simulink model "EMPlanner_cs"  (R2020a)
settings: Solver=ode5  StartTime=0.0  StopTime=55  FixedStep=1/1000  RelTol=1e-3
PreLoadFcn:
  | mbxruntime.callbacks.PreLoadFcn(bdroot);
PostLoadFcn:
  | mbxruntime.callbacks.PostLoadFcn(bdroot);
InitFcn:
  | mbxruntime.callbacks.InitFcn(bdroot);
StartFcn:
  | mbxruntime.callbacks.StartFcn(bdroot);
StopFcn:
  | mbxruntime.callbacks.StopFcn(bdroot);
model workspace: external: MAT-File .\EMPlanner_cs_hws.mat (data not in the file)
values from neighbouring files (symbols this model uses):
  c_factor = 43.75    [emplanner_init.m]
  cf = -175016    [emplanner_init.m]
  control_predict_time = 0.01    [emplanner_init.m]
  cr = -130634    [emplanner_init.m]
  dp_col = 4    [emplanner_init.m]
  dp_row = 9    [emplanner_init.m]
  dp_sample_l = 1    [emplanner_init.m]
  dp_sample_s = 15    [emplanner_init.m]
  dp_w_obs = 1e8    (= 100000000)    [emplanner_init.m]
  dp_w_ref = 20    [emplanner_init.m]
  dp_w_smooth_dddl = 10000    [emplanner_init.m]
  dp_w_smooth_ddl = 2000    [emplanner_init.m]
  dp_w_smooth_dl = 300    [emplanner_init.m]
  KD_PID_distance = 0.0    (= 0)    [emplanner_init.m]
  KD_PID_speed = 0    [emplanner_init.m]
  KI_PID_distance = 0.0    (= 0)    [emplanner_init.m]
  KI_PID_speed = 0    [emplanner_init.m]
  KP_PID_distance = 0.5    [emplanner_init.m]
  KP_PID_speed = 1.8    [emplanner_init.m]
  la = 1.265    [emplanner_init.m]
  lb = 2.947-1.265    (= 1.682)    [emplanner_init.m]
  LQR_K1 = k(:,1)'    [emplanner_init.m]
  LQR_K2 = k(:,2)'    [emplanner_init.m]
  LQR_K3 = k(:,3)'    [emplanner_init.m]
  LQR_K4 = k(:,4)'    [emplanner_init.m]
  m = 2020    [emplanner_init.m]
  path_x = [7.7742 8.77358225507 9.77170536558 10.7685522493 11.7641171228 12.7583983581 13.7513958557 14.7431100776 15.7335416918 16.7226914411 17.7105600952 18.6971484329 ... (551 elements, 551x1)]    [test_path.mat]
  path_y = [-207.8202 -207.82020006 -207.820200616 -207.820202023 -207.82020429 -207.820207237 -207.820210603 -207.820214131 -207.82021762 -207.820220941 -207.820224011 -207.820226778 ... (551 elements, 551x1)]    [test_path.mat]
  qp_referenceline_w_length = 2    [emplanner_init.m]
  qp_referenceline_w_ref = 3    [emplanner_init.m]
  qp_referenceline_w_smooth = 1    [emplanner_init.m]
  qp_referenceline_x_lb = -0.2    [emplanner_init.m]
  qp_referenceline_x_ub = 0.2    [emplanner_init.m]
  qp_referenceline_y_lb = -0.2    [emplanner_init.m]
  qp_referenceline_y_ub = 0.2    [emplanner_init.m]
  rack_displacement = [-39.14 , -37.2 , -35.29 , -33.43 , -31.6 , -29.81 , -28.06 , -26.34 , -24.66 ,      -23.01 , -21.38 , -19.79 , -18.23 , -16.69 , -15.18 , -13.7 , -12.23 , -10.8 , -9.38 , -7.98 ,     -6.61 , -5.25 , -3.91 , -2.59 , -1.29 , 0 , 1.27 , 2.54 , 3.78 , 5.02 , 6.24 , 7.46 , 8.66 ,      9.86 , 11.05 , 12.24 , 13.41 , 14.59 , 15.76 , 16.92 , 18.09 , 19.25 , 20.42 , 21.59 , 22.76 ,      23.93 , 25.11 , 26 ...(+26 chars)    [emplanner_init.m]
  right_wheel_ground = [-70 ,-67.2 , -64.4 , -61.6 , -58.8 , -56 , -53.2 , -50.4 , -47.6 , -44.8 , -42 ,      -39.2 , -36.4 , -33.6 , -30.8 , -28 , -25.2 , -22.4 , -19.6 , -16.8 , -14 , -11.2 , -8.4 , -5.6 ,      -2.8 , 0 , 2.8 , 5.6 , 8.4 , 11.2 , 14 , 16.8 , 19.6 , 22.4 , 25.2 , 28 , 30.8 , 33.6 , 36.4 ,      39.2 , 42 , 44.8 , 47.6 , 50.4 , 53.2 , 56 , 58.8 , 61.6 , 64.4 , 67.2 , 70 ]    [emplanner_init.m]
  vx_break_point = zeros(1,5000)    [emplanner_init.m]
undefined symbols (not defined in the file or in its folder): aubr, DiscIntNeverNeededParam, tablebr, vubr, warningInitialVelocity, x0
libraries: simulink x19, PreScanSimulinkLibrary x12, simulink_extras x5, Solver_SF x1
(part 7 of 9)

== system EMPlanner_cs/Audi_A8_Sedan_2/Dynamics_Simple/ShiftLogic/Detect Increase/Other ==
  In1 : Inport
  Action Port : ActionPort  PropagateVarSize=During execution  ActionPortLabel=else
  Data Type Conversion : DataTypeConversion  OutDataTypeStr=double
  Detect Increase : simulink/Logic and Bit Operations/Detect Increase  vinit=0.0  OutDataTypeStr=uint8
  Out1 : Outport
  wires:
  In1/1 -> Detect Increase/1
  Detect Increase/1 -> Data Type Conversion/1
  Data Type Conversion/1 -> Out1/1

== system EMPlanner_cs/Audi_A8_Sedan_2/Dynamics_Simple/Transmission/Transmission_Ratio/If Action Neutral ==
  In1 : Inport
  Action Port : ActionPort  InitializeStates=reset  PropagateVarSize=During execution  ActionPortLabel=if(u1 == 0)
  Out1 : Outport
  wires:
  In1/1 -> Out1/1

== system EMPlanner_cs/Audi_A8_Sedan_2/Dynamics_Simple/Transmission/Transmission_Ratio/If Action Normal ==
  In1 : Inport
  Action Port : ActionPort  InitializeStates=reset  PropagateVarSize=During execution  ActionPortLabel=else
  Out1 : Outport
  wires:
  In1/1 -> Out1/1

== system EMPlanner_cs/Audi_A8_Sedan_2/Dynamics_Simple/Transmission/Transmission_Ratio/If Action Reverse ==
  In1 : Inport
  Action Port : ActionPort  InitializeStates=reset  PropagateVarSize=During execution  ActionPortLabel=elseif(u1 == -1)
  Reverse : Gain  Gain=-1
  Out1 : Outport
  wires:
  Reverse/1 -> Out1/1
  In1/1 -> Reverse/1

== system EMPlanner_cs/Audi_A8_Sedan_2/PathFollower_Preview_1/LateralController/SteeringWheelAngle/FirstOrderDynamics ==
  In : Inport
  TimeConstant[s] : Inport  Port=2
  Reset : Inport  Port=3
  x0 : Inport  Port=4
  1|TimeConstant : Product  Inputs=*/  InputSameDT=on  SaturateOnIntegerOverflow=on  OutDataTypeStr=Inherit: Same as first input
  Discrete-Time Integrator : DiscreteIntegrator  ExternalReset=rising  InitialConditionSource=external  InitialCondition=x0  SampleTime=CSSampleTime  ICPrevOutput=DiscIntNeverNeededParam  ICPrevScaledInput=DiscIntNeverNeededParam
  IC : InitialCondition  Value=0
  Saturation : Saturate  UpperLimit=1e300  LowerLimit=0.001
  Sum : Sum  Inputs=-+|  InputSameDT=on  SaturateOnIntegerOverflow=on  OutDataTypeStr=Inherit: Same as first input
  Out : Outport
  wires:
  IC/1 -> Discrete-Time Integrator/3
  In/1 -> Sum/2
  x0/1 -> IC/1
  Reset/1 -> Discrete-Time Integrator/2
  1|TimeConstant/1 -> Discrete-Time Integrator/1
  Sum/1 -> 1|TimeConstant/1
  Saturation/1 -> 1|TimeConstant/2
  TimeConstant[s]/1 -> Saturation/1
  Discrete-Time Integrator/1 -> Out/1, Sum/1

== system EMPlanner_cs/Audi_A8_Sedan_2/PathFollower_Preview_1/LateralController/SteeringWheelAngle/Sat_Total ==
  In : Inport
  Sat_Limit : Inport  Port=2
  Gain1 : Gain  Gain=-1  SaturateOnIntegerOverflow=on  OutDataTypeStr=Inherit: Same as input  ParamDataTypeStr=Inherit: Same as input
  RelOp_UL : RelationalOperator  RndMeth=Nearest
  RelOp_UL1 : RelationalOperator  Operator=<=  RndMeth=Nearest
  Sum : Sum  Inputs=++|  SaturateOnIntegerOverflow=on
  Switch : Switch  Threshold=0.5  SaturateOnIntegerOverflow=on
  Switch1 : Switch  Threshold=0.5  SaturateOnIntegerOverflow=on
  Sat_Total : Outport
  Sat_Info : Outport  Port=2
  wires:
  Sat_Limit/1 -> Gain1/1, Switch/1, RelOp_UL/2
  RelOp_UL/1 -> Switch/2, Sum/2
  Switch/1 -> RelOp_UL1/1, Switch1/3
  Gain1/1 -> RelOp_UL1/2, Switch1/1
  RelOp_UL1/1 -> Switch1/2, Sum/1
  In/1 -> Switch/3, RelOp_UL/1
  Switch1/1 -> Sat_Total/1
  Sum/1 -> Sat_Info/1

== system EMPlanner_cs/Audi_A8_Sedan_2/PathFollower_Preview_1/LongitudinalController/If Desired Velocity ~= 0/PID_AWU ==
  e : Inport
  Derivative Gain : Gain  Gain=D  SaturateOnIntegerOverflow=on  OutDataTypeStr=Inherit: Same as input  ParamDataTypeStr=Inherit: Same as input
  Discrete-Time Integrator : DiscreteIntegrator  gainval=1  SampleTime=CSSampleTime  UpperSaturationLimit=100  LowerSaturationLimit=-100  ICPrevOutput=DiscIntNeverNeededParam  ICPrevScaledInput=DiscIntNeverNeededParam
  Filter : DiscreteIntegrator  gainval=1  SampleTime=CSSampleTime  ICPrevOutput=DiscIntNeverNeededParam  ICPrevScaledInput=DiscIntNeverNeededParam
  Integral Gain : Gain  Gain=I  SaturateOnIntegerOverflow=on  OutDataTypeStr=Inherit: Same as input  ParamDataTypeStr=Inherit: Same as input
  Integral Gain1 : Gain  Gain=LongCtrl_AWU  SaturateOnIntegerOverflow=on  OutDataTypeStr=Inherit: Same as input  ParamDataTypeStr=Inherit: Same as input
  Proportional Gain : Gain  Gain=P  SaturateOnIntegerOverflow=on  OutDataTypeStr=Inherit: Same as input  ParamDataTypeStr=Inherit: Same as input
  Saturation : Saturate  UpperLimit=100  LowerLimit=-100
  Sum : Sum  Inputs=+++  InputSameDT=on  SaturateOnIntegerOverflow=on  OutDataTypeStr=Inherit: Same as first input
  Sum1 : Sum  Inputs=|+-  InputSameDT=on  SaturateOnIntegerOverflow=on  OutDataTypeStr=Inherit: Same as first input
  Sum2 : Sum  Inputs=|++  InputSameDT=on  SaturateOnIntegerOverflow=on  OutDataTypeStr=Inherit: Same as first input
  Sum3 : Sum  Inputs=-+|  InputSameDT=on  SaturateOnIntegerOverflow=on  OutDataTypeStr=Inherit: Same as first input
  u : Outport  InitialOutput=0
  wires:
  Integral Gain1/1 -> Sum2/2
  Sum3/1 -> Integral Gain1/1
  Saturation/1 -> Sum3/2, u/1
  Sum2/1 -> Discrete-Time Integrator/1
  Sum1/1 -> Sum/3, Filter/1
  Filter/1 -> Sum1/2
  Derivative Gain/1 -> Sum1/1
  Sum/1 -> Sum3/1, Saturation/1
  e/1 -> Integral Gain/1, Proportional Gain/1, Derivative Gain/1
  Discrete-Time Integrator/1 -> Sum/2
  Proportional Gain/1 -> Sum/1
  Integral Gain/1 -> Sum2/1

== system EMPlanner_cs/Audi_A8_Sedan_2/Dynamics_Simple/Chassis/Bicycle_model_[XYZ]/X_Motion/Air&RoadResistance ==
  vx_[ms-1] : Inport
  Gain : Gain  Gain=1/p.Rw
  Road & Aerodyn Resistances : Fcn  Expr=p.Rroad + p.Rair*u^2
  Saturation1 : Saturate  UpperLimit=5/15  LowerLimit=-5/15
  Sign : Signum
  "[ms-1] 2 [rads-1]" : Gain  Gain=1/p.Rw  SaturateOnIntegerOverflow=on  OutDataTypeStr=Inherit: Same as input  ParamDataTypeStr=Inherit: Same as input
  signed load1 : Product  InputSameDT=on  SaturateOnIntegerOverflow=on  OutDataTypeStr=Inherit: Same as first input
  Resistance_Force : Outport
  wires:
  signed load1/1 -> Resistance_Force/1  "F_[N]"
  vx_[ms-1]/1 -> Road & Aerodyn Resistances/1, "[ms-1] 2 [rads-1]"/1
  Saturation1/1 -> Sign/1
  "[ms-1] 2 [rads-1]"/1 -> Saturation1/1
  Road & Aerodyn Resistances/1 -> Gain/1  "ResistanceTorque_[Nm]"
  Sign/1 -> signed load1/2  "sign"
  Gain/1 -> signed load1/1  "Resistance Force_[N]"

== system EMPlanner_cs/Audi_A8_Sedan_2/Dynamics_Simple/Chassis/Bicycle_model_[XYZ]/X_Motion/BrakeSystem ==
  vx_[ms-1] : Inport
  BrakePressure_[bar] : Inport  Port=2
  Gain : Gain  Gain=1/p.Rw
  Saturation : Saturate  UpperLimit=p.PBrakeMax  LowerLimit=0
  Saturation1 : Saturate  UpperLimit=5/15  LowerLimit=-5/15
  Sign : Signum
  "[ms-1] 2 [rads-1]" : Gain  Gain=1/p.Rw  SaturateOnIntegerOverflow=on  OutDataTypeStr=Inherit: Same as input  ParamDataTypeStr=Inherit: Same as input
  braking Q factor : Gain  Gain=p.Qfac  SaturateOnIntegerOverflow=on  OutDataTypeStr=Inherit: Same as input  ParamDataTypeStr=Inherit: Same as input
  signed load1 : Product  InputSameDT=on  SaturateOnIntegerOverflow=on  OutDataTypeStr=Inherit: Same as first input
  BrakeForce : Outport
  BrakeTorqueAbs : Outport  Port=2
  wires:
  braking Q factor/1 -> BrakeTorqueAbs/1, Gain/1
  BrakePressure_[bar]/1 -> Saturation/1
  Saturation/1 -> braking Q factor/1
  vx_[ms-1]/1 -> "[ms-1] 2 [rads-1]"/1
  Saturation1/1 -> Sign/1
  "[ms-1] 2 [rads-1]"/1 -> Saturation1/1
  Sign/1 -> signed load1/2  "sign"
  signed load1/1 -> BrakeForce/1
  Gain/1 -> signed load1/1

== system EMPlanner_cs/Audi_A8_Sedan_2/Dynamics_Simple/Chassis/Bicycle_model_[XYZ]/X_Motion/Configurable Subsystem ==
  In1 : Inport
  In2 : Inport  Port=2
  In3 : Inport  Port=3
  Integrator : Integrator  ExternalReset=level  InitialConditionSource=external
  Out1 : Outport
  wires:
  In1/1 -> Integrator/1
  In2/1 -> Integrator/2
  In3/1 -> Integrator/3
  Integrator/1 -> Out1/1

== system EMPlanner_cs/Audi_A8_Sedan_2/Dynamics_Simple/Chassis/Bicycle_model_[XYZ]/X_Motion/Configurable Subsystem1 ==
  In1 : Inport
  Torsional damping : TransferFcn  Denominator=[0.1 1]
  Out1 : Outport
  wires:
  In1/1 -> Torsional damping/1
  Torsional damping/1 -> Out1/1

== system EMPlanner_cs/Audi_A8_Sedan_2/Dynamics_Simple/Chassis/Bicycle_model_[XYZ]/X_Motion/Max RPM and zero- velocity detection ==
  note: Set to zero after infinite small time-step
  note: Zero velocity detection
  ax : Inport
  Drive Torque : Inport  Port=2
  Brake Torque : Inport  Port=3
  v0 : Inport  Port=4
  vx : Inport  Port=5
  Abs : Abs
  Abs1 : Abs
  Compare To Zero : simulink/Logic and Bit Operations/Compare To Zero  relop=<=  OutDataTypeStr=boolean  ZeroCross=off
  Compare To Zero1 : simulink/Logic and Bit Operations/Compare To Zero  relop=>=  OutDataTypeStr=boolean  ZeroCross=off
  Compare To Zero2 : simulink/Logic and Bit Operations/Compare To Zero  relop=>=  OutDataTypeStr=boolean  ZeroCross=off
  Compare To Zero3 : simulink/Logic and Bit Operations/Compare To Zero  relop=<=  OutDataTypeStr=boolean  ZeroCross=off
  Configurable Subsystem : Subsystem  BlockChoice=Step  mask{ComputationMode=ComputationMode}
      mask prompts: ComputationMode "Compuation mode:"
      mask init:
      | SetComputationMode(gcb,ComputationMode);
      settings: AttributesFormatString=%<BlockChoice>  OpenFcn=BringToFront(gcb);  MemberBlocks=Discrete Step,Step
      settings: TemplateBlock=|
      | PreScanSimulinkLibrary/Configurable Subsystems/Step Function/Configurable
      | Subsystem
  Constant : Constant
  Constant1 : Constant
  Logical Operator : Logic  AllPortsSameDT=off  OutDataTypeStr=boolean
  Logical Operator1 : Logic  AllPortsSameDT=off  OutDataTypeStr=boolean
  Logical Operator2 : Logic  Operator=NOT  AllPortsSameDT=off  OutDataTypeStr=boolean
  Logical Operator3 : Logic  AllPortsSameDT=off  OutDataTypeStr=boolean
  Logical Operator4 : Logic  Operator=OR  AllPortsSameDT=off  OutDataTypeStr=boolean
  Memory : Memory
  Memory1 : Memory
  Memory2 : Memory
  Product : Product  RndMeth=Zero
  Relational Operator : RelationalOperator  Operator=<  OutDataTypeStr=boolean  RndMeth=Nearest
  SR-Memory : Subsystem
  Sum : Sum  Inputs=|-+
  Switch : Switch  Criteria=u2 ~= 0  Threshold=0.5
  ax is 0 : Constant  Value=0
  ax_out : Outport
  vx_reset : Outport  Port=2
  x0 : Outport  Port=3
  wires:
  Logical Operator4/1 -> Logical Operator1/1
  vx/1 -> Compare To Zero/1, Compare To Zero2/1, Memory2/1, Memory/1  "vx"
  Memory2/1 -> Compare To Zero3/1
  Compare To Zero2/1 -> Logical Operator3/1
  Compare To Zero3/1 -> Logical Operator3/2
  Logical Operator3/1 -> Logical Operator4/2  "zero-crossing backward"
  Memory/1 -> Compare To Zero1/1
  Compare To Zero/1 -> Logical Operator/1
  Compare To Zero1/1 -> Logical Operator/2
  Logical Operator/1 -> Logical Operator4/1  "zero-crossing forward"
  Abs/1 -> Relational Operator/1
  Abs1/1 -> Relational Operator/2
  Drive Torque/1 -> Abs/1
  Brake Torque/1 -> Abs1/1
  Relational Operator/1 -> Logical Operator1/2, Logical Operator2/1
  Logical Operator1/1 -> SR-Memory/2(Set)
  Constant/1 -> SR-Memory/1(Signal)
  Logical Operator2/1 -> SR-Memory/3(Reset)
  SR-Memory/1(Out) -> Sum/1, Memory1/1
  Switch/1 -> ax_out/1
  Sum/1 -> Switch/2
  ax is 0/1 -> Switch/3
  Constant1/1 -> Sum/2
  v0/1 -> Product/1
  Product/1 -> x0/1
  Configurable Subsystem/1(Out1) -> Product/2
  ax/1 -> Switch/1  "ax"
  Memory1/1 -> vx_reset/1  "vx"

== system EMPlanner_cs/Audi_A8_Sedan_2/Dynamics_Simple/Chassis/Bicycle_model_[XYZ]/Y & Yaw_Motion/Configurable Subsystem ==
  In1 : Inport
  In2 : Inport  Port=2
  Integrator : Integrator  ExternalReset=level
  Out1 : Outport
  wires:
  In1/1 -> Integrator/1
  In2/1 -> Integrator/2
  Integrator/1 -> Out1/1

== system EMPlanner_cs/Audi_A8_Sedan_2/Dynamics_Simple/Chassis/Bicycle_model_[XYZ]/Y & Yaw_Motion/Configurable Subsystem1 ==
  In1 : Inport
  Integrator : Integrator
  Out1 : Outport
  wires:
  In1/1 -> Integrator/1
  Integrator/1 -> Out1/1

== system EMPlanner_cs/Audi_A8_Sedan_2/Dynamics_Simple/Chassis/Bicycle_model_[XYZ]/Y & Yaw_Motion/Configurable Subsystem2 ==
  In1 : Inport
  In2 : Inport  Port=2
  Integrator : Integrator  ExternalReset=level
  Out1 : Outport
  wires:
  In1/1 -> Integrator/1
  In2/1 -> Integrator/2
  Integrator/1 -> Out1/1

== system EMPlanner_cs/Audi_A8_Sedan_2/Dynamics_Simple/Chassis/Bicycle_model_[XYZ]/Z, Pitch_Motion & Roll_Motion/Configurable Subsystem ==
  In1 : Inport
  Integrator : Integrator  LimitOutput=on  UpperSaturationLimit=5*pi/180  LowerSaturationLimit=-5*pi/180
  Out1 : Outport
  wires:
  In1/1 -> Integrator/1
  Integrator/1 -> Out1/1

== system EMPlanner_cs/Audi_A8_Sedan_2/Dynamics_Simple/Chassis/Bicycle_model_[XYZ]/Z, Pitch_Motion & Roll_Motion/Configurable Subsystem1 ==
  In1 : Inport
  Integrator : Integrator
  Out1 : Outport
  wires:
  In1/1 -> Integrator/1
  Integrator/1 -> Out1/1

== system EMPlanner_cs/Audi_A8_Sedan_2/Dynamics_Simple/Chassis/Bicycle_model_[XYZ]/Z, Pitch_Motion & Roll_Motion/Configurable Subsystem2 ==
  In1 : Inport
  Integrator : Integrator
  Out1 : Outport
  wires:
  In1/1 -> Integrator/1
  Integrator/1 -> Out1/1

== system EMPlanner_cs/Audi_A8_Sedan_2/Dynamics_Simple/Chassis/Bicycle_model_[XYZ]/Z, Pitch_Motion & Roll_Motion/Configurable Subsystem3 ==
  In1 : Inport
  Integrator : Integrator
  Out1 : Outport
  wires:
  In1/1 -> Integrator/1
  Integrator/1 -> Out1/1

== system EMPlanner_cs/Audi_A8_Sedan_2/Dynamics_Simple/Chassis/Bicycle_model_[XYZ]/Z, Pitch_Motion & Roll_Motion/Configurable Subsystem4 ==
  In1 : Inport
  Integrator : Integrator
  Out1 : Outport
  wires:
  In1/1 -> Integrator/1
  Integrator/1 -> Out1/1

== system EMPlanner_cs/Audi_A8_Sedan_2/Dynamics_Simple/Chassis/Bicycle_model_[XYZ]/Z, Pitch_Motion & Roll_Motion/Configurable Subsystem5 ==
  In1 : Inport
  Integrator : Integrator
  Out1 : Outport
  wires:
  In1/1 -> Integrator/1
  Integrator/1 -> Out1/1

== system EMPlanner_cs/Audi_A8_Sedan_2/Dynamics_Simple/Chassis/Bicycle_model_[XYZ]/Z, Pitch_Motion & Roll_Motion/Configurable Subsystem9 ==
  In1 : Inport
  Derivative : Derivative
  Out1 : Outport
  wires:
  In1/1 -> Derivative/1
  Derivative/1 -> Out1/1

== system EMPlanner_cs/Audi_A8_Sedan_2/Dynamics_Simple/Chassis/FrontTyre/AlphaFront/Enabled Subsystem ==
  In : Inport
  Enable : EnablePort  PropagateVarSize=During execution
  AlphaFront : Fcn  Expr=-atan( (u(2)+u(3)*p.a)/u(1) )
  Alpha : Outport  OutputWhenDisabled=reset  InitialOutput=[0]
  wires:
  AlphaFront/1 -> Alpha/1
  In/1 -> AlphaFront/1

== system EMPlanner_cs/Audi_A8_Sedan_2/Dynamics_Simple/Chassis/RearTyre/AlphaRear/Enabled Subsystem ==
  In : Inport
  Enable : EnablePort  PropagateVarSize=During execution
  AlphaRear : Fcn  Expr=-atan( (u(2)-u(3)*p.b)/u(1) )
  Alpha : Outport  OutputWhenDisabled=reset  InitialOutput=[0]
  wires:
  AlphaRear/1 -> Alpha/1
  In/1 -> AlphaRear/1

== system EMPlanner_cs/Audi_A8_Sedan_2/Dynamics_Simple/Chassis/Bicycle_model_[XYZ]/X_Motion/Max RPM and zero- velocity detection/Configurable Subsystem ==
  Step : Step  Time=0.0001  Before=1  After=0  SampleTime=0
  Out1 : Outport
  wires:
  Step/1 -> Out1/1

== system EMPlanner_cs/Audi_A8_Sedan_2/Dynamics_Simple/Chassis/Bicycle_model_[XYZ]/X_Motion/Max RPM and zero- velocity detection/SR-Memory ==
  Signal : Inport
  Set : Inport  Port=2
  Reset : Inport  Port=3
  Constant : Constant  Value=0
  Detect Rise Positive : simulink/Logic and Bit Operations/Detect Rise Positive  vinit=0  OutDataTypeStr=uint8
  Detect Rise Positive1 : simulink/Logic and Bit Operations/Detect Rise Positive  vinit=0  OutDataTypeStr=uint8
  Manual Switch : ManualSwitch
  Manual Switch1 : ManualSwitch
  Switch : Switch  Criteria=u2 ~= 0
  Switch1 : Switch  Criteria=u2 ~= 0
  Unit Delay : UnitDelay  SampleTime=-1  HasFrameUpgradeWarning=on
  Out : Outport
  wires:
  Constant/1 -> Switch1/1
  Switch/1 -> Switch1/3
  Switch1/1 -> Unit Delay/1, Out/1
  Manual Switch1/1 -> Switch1/2
  Reset/1 -> Manual Switch1/2, Detect Rise Positive1/1
  Detect Rise Positive1/1 -> Manual Switch1/1
  Signal/1 -> Switch/1
  Unit Delay/1 -> Switch/3
  Set/1 -> Detect Rise Positive/1, Manual Switch/2
  Detect Rise Positive/1 -> Manual Switch/1
  Manual Switch/1 -> Switch/2

== matlab function EMPlanner_cs/Audi_A8_Sedan_1/decision&planning module/EM Planner/calc plan start info and stitch trajectory ==
  data: pre_planPath_x_set_gcs input; plan_startPoint_x_gcs output; pre_planPath_y_set_gcs input; pre_planPath_heading_set_gcs input; pre_planPath_kappa_set_gcs input; pre_planPath_velocity_set_gcs input; pre_planPath_acceleration_set_gcs input; pre_planPath_time_set input; current_time input; host_x_gcs input; host_y_gcs input; host_heading_gcs input; host_vx_vcs input; host_vy_vcs input; host_ax_vcs input; host_ay_vcs input; plan_startPoint_y_gcs output; plan_startPoint_heading_gcs output; plan_startPoint_kappa_gcs output; plan_startPoint_vx_gcs output; plan_startPoint_vy_gcs output; plan_startPoint_ax_gcs output; plan_startPoint_ay_gcs output; plan_startPoint_time output; stitchPath_x_set_gcs output; stitchPath_y_set_gcs output; stitchPath_heading_set_gcs output; stitchPath_kappa_set_gcs output; stitchPath_velocity_set_gcs output; stitchPath_acceleration_set_gcs output; stitchPath_time_set output; host_dheading_gcs input
function [plan_startPoint_x_gcs,plan_startPoint_y_gcs,plan_startPoint_heading_gcs,plan_startPoint_kappa_gcs, ...
    plan_startPoint_vx_gcs,plan_startPoint_vy_gcs,plan_startPoint_ax_gcs,plan_startPoint_ay_gcs,plan_startPoint_time,...
    stitchPath_x_set_gcs,stitchPath_y_set_gcs,stitchPath_heading_set_gcs,stitchPath_kappa_set_gcs,stitchPath_velocity_set_gcs,...
    stitchPath_acceleration_set_gcs,stitchPath_time_set] = fun(pre_planPath_x_set_gcs,pre_planPath_y_set_gcs,...
    pre_planPath_heading_set_gcs,pre_planPath_kappa_set_gcs,pre_planPath_velocity_set_gcs,pre_planPath_acceleration_set_gcs,...
    pre_planPath_time_set,current_time,host_x_gcs,host_y_gcs,host_heading_gcs,host_vx_vcs,host_vy_vcs,host_ax_vcs,host_ay_vcs,host_dheading_gcs)
% 该函数将计算规划起点和待拼接轨迹的信息
% plan_startPoint_x_gcs,plan_startPoint_y_gcs,plan_startPoint_heading_gcs,plan_startPoint_kappa_gcs,plan_startPoint_vx_gcs
% plan_startPoint_vy_gcs,plan_startPoint_ax_gcs,plan_startPoint_ay_gcs,plan_startPoint_time 规划起点信息
% stitchPath_x_set_gcs,stitchPath_y_set_gcs,stitchPath_heading_set_gcs,stitchPath_kappa_set_gcs,
% stitchPath_velocity_set_gcs,stitchPath_acceleration_set_gcs,stitchPath_time_set 待拼接轨迹信息
% pre_planPath_x_set_gcs,pre_planPath_y_set_gcs,pre_planPath_heading_set_gcs,pre_planPath_kappa_set_gcs,
% pre_planPath_velocity_set_gcs,pre_planPath_acceleration_set_gcs,pre_planPath_time_set 上个周期规划轨迹信息
% current_time 当前时间
% host_x_gcs,host_y_gcs,host_heading_gcs,host_vx_vcs,host_vy_vcs,host_ax_vcs,host_ay_vcs 自车当前时间信息

% 对输出进行初始化
% 假设取规划起点前面的20个点作为待拼接轨迹 对其初始化
n = 20;
stitchPath_x_set_gcs = zeros(n,1);stitchPath_y_set_gcs = zeros(n,1); stitchPath_heading_set_gcs = zeros(n,1);
stitchPath_kappa_set_gcs = zeros(n,1); stitchPath_velocity_set_gcs = zeros(n,1); stitchPath_acceleration_set_gcs = zeros(n,1);
stitchPath_time_set = ones(n,1) * -1; %时间为负代表没有对应的拼接轨迹
dt = 0.1; % 规划周期100ms 0.1s
persistent is_first_run;
% 得到车辆的x方向和y方向的速度和加速度
host_vx_gcs = host_vx_vcs * cos(host_heading_gcs) - host_vy_vcs * sin(host_heading_gcs);
host_vy_gcs = host_vx_vcs * sin(host_heading_gcs) + host_vy_vcs * cos(host_heading_gcs);
host_ax_gcs = host_ax_vcs * cos(host_heading_gcs) - host_ay_vcs * sin(host_heading_gcs);
host_ay_gcs = host_ax_vcs * sin(host_heading_gcs) + host_ay_vcs * cos(host_heading_gcs);
if isempty(is_first_run)
    is_first_run = 0;
    % 第一次运行 没有上周期轨迹  无需拼接  通过车辆动力学递推dt时间之后的信息作为规划起点 假设dt时间做匀加速运动
    plan_startPoint_x_gcs = host_x_gcs + host_vx_gcs * dt + 0.5 * host_ax_gcs * dt^2;
    plan_startPoint_y_gcs = host_y_gcs + host_vy_gcs * dt + 0.5 * host_ay_gcs * dt^2;
    plan_startPoint_heading_gcs = host_heading_gcs + host_dheading_gcs * dt;
    plan_startPoint_kappa_gcs = 0;
    plan_startPoint_vx_gcs = host_vx_gcs + host_ax_gcs * dt;
    plan_startPoint_vy_gcs = host_vy_gcs + host_ay_gcs * dt;
    plan_startPoint_ax_gcs = host_ax_gcs;
    plan_startPoint_ay_gcs = host_ay_gcs;
    plan_startPoint_time = current_time + dt;
else
    % 后续运行  有上周期轨迹 
    % 判断自身是否跟上上周期规划轨迹 如果没有跟上 无需拼接
    % 首先求出上周期自车应该在的位置
    for i = 1:length(pre_planPath_time_set)-1
        if current_time >= pre_planPath_time_set(i) && current_time < pre_planPath_time_set(i+1)
            break;
        end
    end
    % 当前时间current_time对应上周期规划轨迹i时刻位置
    % 提取上周期规划本车信息
    pre_host_x_gcs = pre_planPath_x_set_gcs(i); pre_host_y_gcs = pre_planPath_y_set_gcs(i);
    pre_host_heading_gcs = pre_planPath_heading_set_gcs(i);
    % 计算本周期本车信息和上周期规划本车信息的横向误差和纵向误差
    vector_preHost_curHost = [host_x_gcs,host_y_gcs] - [pre_host_x_gcs,pre_host_y_gcs];
    vector_tor_preHost = [cos(pre_host_heading_gcs),sin(pre_host_heading_gcs)];
    vector_nor_preHost = [-sin(pre_host_heading_gcs),cos(pre_host_heading_gcs)];
    lat_er = dot(vector_preHost_curHost,vector_tor_preHost);
    long_er = dot(vector_preHost_curHost,vector_nor_preHost);
    if abs(lat_er) > 0.5 || abs(long_er) > 2.5
        % 如果横向误差大于0.5或纵向误差大于2.5 视为车辆控制没有跟上规划
        % 无需拼接轨迹  通过车辆动力学递推dt时间之后的信息作为规划起点 假设dt时间做匀加速运动
        plan_startPoint_x_gcs = host_x_gcs + host_vx_gcs * dt + 0.5 * host_ax_gcs * dt^2;
        plan_startPoint_y_gcs = host_y_gcs + host_vy_gcs * dt + 0.5 * host_ay_gcs * dt^2;
        plan_startPoint_heading_gcs = host_heading_gcs + host_dheading_gcs * dt;
        plan_startPoint_kappa_gcs = 0;
        plan_startPoint_vx_gcs = host_vx_gcs + host_ax_gcs * dt;
        plan_startPoint_vy_gcs = host_vy_gcs + host_ay_gcs * dt;
        plan_startPoint_ax_gcs = host_ax_gcs;
        plan_startPoint_ay_gcs = host_ay_gcs;
        plan_startPoint_time = current_time + dt;
    else
        % 车辆控制跟上规划 需要拼接轨迹
        % 首先计算current_time+dt时刻对应上周期规划轨迹j时刻位置 作为规划起点
        for j = i:length(pre_planPath_time_set)-1
            if current_time+dt >= pre_planPath_time_set(j) && current_time+dt < pre_planPath_time_set(j+1)
                break;
            end
        end
        % 提取上周期规划轨迹j时刻位置信息作为规划起点信息
        plan_startPoint_x_gcs = pre_planPath_x_set_gcs(j);
        plan_startPoint_y_gcs = pre_planPath_y_set_gcs(j);
        plan_startPoint_heading_gcs = pre_planPath_heading_set_gcs(j);
        plan_startPoint_kappa_gcs = pre_planPath_kappa_set_gcs(j);
        % 需要注意的是pre_planPath_velocity_set_gcs(j) 规划路径的速度为沿路径的切向速度 需要分解
        plan_startPoint_vx_gcs = pre_planPath_velocity_set_gcs(j) * cos(pre_planPath_heading_set_gcs(j));
        plan_startPoint_vy_gcs = pre_planPath_velocity_set_gcs(j) * sin(pre_planPath_heading_set_gcs(j));
        % 需要注意的是pre_planPath_acceleration_set_gcs(j) 规划路径的加速度为沿路径的切向加速度 实际上还有法向加速度 
        % 需要先求出法向加速度 再进行求解  an = v^2/R = v^2*k
        % 将加速度转化成向量 这样可以直接包括方向
        tor = [cos(pre_planPath_heading_set_gcs(j)),sin(pre_planPath_heading_set_gcs(j))];
        nor = [-sin(pre_planPath_heading_set_gcs(j)),cos(pre_planPath_heading_set_gcs(j))];
        a_tor = pre_planPath_acceleration_set_gcs(j) * tor;
        a_nor = pre_planPath_velocity_set_gcs(j)^2 * pre_planPath_kappa_set_gcs(j) * nor;
        % 通过向量进行分解 向量都可以看成是绝对x方向和绝对y方向组成 
        plan_startPoint_ax_gcs = a_tor(1) + a_nor(1);
        plan_startPoint_ay_gcs = a_tor(2) + a_nor(2);
        plan_startPoint_time = pre_planPath_time_set(j);
        % 选取规划起点前面的20个点作为待拼接轨迹
        if j > 20
            % 第一种情况 规划起点前面的点够20个
            start_index = j - 20;
            stitchPath_x_set_gcs(1:n) = pre_planPath_x_set_gcs(start_index:start_index+19);
            stitchPath_y_set_gcs(1:n) = pre_planPath_y_set_gcs(start_index:start_index+19);
            stitchPath_heading_set_gcs(1:n) = pre_planPath_heading_set_gcs(start_index:start_index+19);
            stitchPath_kappa_set_gcs(1:n) = pre_planPath_kappa_set_gcs(start_index:start_index+19);
            stitchPath_velocity_set_gcs(1:n) = pre_planPath_velocity_set_gcs(start_index:start_index+19);
            stitchPath_acceleration_set_gcs(1:n) = pre_planPath_acceleration_set_gcs(start_index:start_index+19);
            stitchPath_time_set(1:n) = pre_planPath_time_set(start_index:start_index+19);
        else
            % 第二种情况 规划起点前面的点不够20个
            start_index = 1;
            % 优先填充后面的点
            stitchPath_x_set_gcs(n-(j-2):n) = pre_planPath_x_set_gcs(start_index:j-1);
            stitchPath_y_set_gcs(n-(j-2):n) = pre_planPath_y_set_gcs(start_index:j-1);
            stitchPath_heading_set_gcs(n-(j-2):n) = pre_planPath_heading_set_gcs(start_index:j-1);
            stitchPath_kappa_set_gcs(n-(j-2):n) = pre_planPath_kappa_set_gcs(start_index:j-1);
            stitchPath_velocity_set_gcs(n-(j-2):n) = pre_planPath_velocity_set_gcs(start_index:j-1);
            stitchPath_acceleration_set_gcs(n-(j-2):n) = pre_planPath_acceleration_set_gcs(start_index:j-1);
            stitchPath_time_set(n-(j-2):n) = pre_planPath_time_set(start_index:j-1);
        end
    end
end
end

== matlab function EMPlanner_cs/Audi_A8_Sedan_1/decision&planning module/referenceline provider/MATLAB Function4 ==
  data: path_x_init_set_gcs input; path_x_set_gcs output; path_y_init_set_gcs input; w_smooth input; w_length input; w_ref input; x_lb input; x_ub input; y_lb input; y_ub input; path_y_set_gcs output
function [path_x_set_gcs,path_y_set_gcs] = fun(path_x_init_set_gcs, path_y_init_set_gcs,w_smooth,w_length,w_ref,...
    x_lb,x_ub,y_lb,y_ub)
% 该函数将通过二次规划方法平滑给定路径
% path_x_init_set_gcs, path_x_init_set_gcs 待平滑轨迹点信息
% w_smooth,w_length,w_ref 二次规划权重 平滑权重 紧凑权重(平滑之后尽可能长度短) 相似权重(与之前路径尽可能接近)
% x_lb,x_ub,y_lb,y_ub 平滑之后x,y坐标上下限

% 需要利用上周期平滑前轨迹信息和平滑后轨迹信息  因此需要定义静态变量来保存
% 如果本周期平滑前轨迹信息和上周期平滑前轨迹一模一样 就无需平滑
persistent is_first_run;
persistent pre_path_x_init_set_gcs; persistent pre_path_y_init_set_gcs; 
persistent pre_path_x_set_gcs; persistent pre_path_y_set_gcs; 

if isempty(is_first_run)
    is_first_run = 0;
    % 第一次 无需判断 需要平滑 调用二次规划平滑路径函数
    [path_x_set_gcs,path_y_set_gcs] = QpSmoothPath(path_x_init_set_gcs,path_y_init_set_gcs,...
    w_smooth,w_length,w_ref,x_lb,x_ub,y_lb,y_ub);
    % 保存该周期结果 供下周期使用
    pre_path_x_init_set_gcs = path_x_init_set_gcs; pre_path_y_init_set_gcs = path_y_init_set_gcs;
    pre_path_x_set_gcs = path_x_set_gcs; pre_path_y_set_gcs = path_y_set_gcs;
else
    % 判断本周期平滑前轨迹信息和上周期平滑前轨迹是否一模一样 判断起点就可以 因为采样点往后都是一样的
    if pre_path_x_init_set_gcs(1) == path_x_init_set_gcs(1) && pre_path_x_init_set_gcs(2) == path_x_init_set_gcs(2)
        % 无需平滑 直接采用上周期平滑结果即可
        path_x_set_gcs = pre_path_x_set_gcs; path_y_set_gcs = pre_path_y_set_gcs;
    else
        % 重新平滑
        [path_x_set_gcs,path_y_set_gcs] = QpSmoothPath(path_x_init_set_gcs,path_y_init_set_gcs,...
                                                        w_smooth,w_length,w_ref,x_lb,x_ub,y_lb,y_ub);
    end
     % 保存该周期结果 供下周期使用
     pre_path_x_init_set_gcs = path_x_init_set_gcs; pre_path_y_init_set_gcs = path_y_init_set_gcs;
     pre_path_x_set_gcs = path_x_set_gcs; pre_path_y_set_gcs = path_y_set_gcs;
end
end

== matlab function EMPlanner_cs/Audi_A8_Sedan_1/control module2/MATLAB Function ==
  data: trajectory_x input; xr output; trajectory_y input; trajectory_heading input; trajectory_kappa input; trajectory_speed input; trajectory_accel input; trajectory_time input; current_time input; yr output; thetar output; kappar output; vr output; ar output
function [xr,yr,thetar,kappar,vr,ar] = fcn(trajectory_x,trajectory_y,trajectory_heading,...
    trajectory_kappa,trajectory_speed,trajectory_accel,trajectory_time,current_time)
% 该函数根据规划的轨迹计算出期望跟踪的点
% 由于控制也是有延迟，所以控制发出的期望跟踪的点是current_time + 0.01;
control_time = current_time + 0.01;
% 规划发出的轨迹有一部分是拼接的，在刚启动的时候，stitch_time = -1,因此要先把它去掉
start_index = 1;
while (trajectory_time(start_index) == -1)
    start_index = start_index + 1;
end
% 使用interp1插值计算得到xr yr thetar,kappar,vr,ar
% 由于interp1在端点会得到nan，因此需要防一手
% 解释，为什么需要trajectory_time(start_index) ~= 0
% 因为在刚启动时规划先执行(100ms)，当规划完毕的时候控制已经执行了10次
% 那么在最开始的时候，规划还没给结果是控制已经执行了10次，在这10次中控制跟踪的轨迹是空轨迹
% simulink 空轨迹表示为 0，0，0，0，0，0......,这样trajectory_time
% 也全是0，trajectory_time不单调递增
% 而interp1(x,y,x0)要求x必须要单调递增，否则会报错，所以当规划首次运行时控制需要执行下面这个else分支的代码，否则会报错
if control_time > trajectory_time(start_index) && trajectory_time(start_index) ~= 0
    xr = interp1(trajectory_time(start_index:end),trajectory_x(start_index:end),control_time);
    yr = interp1(trajectory_time(start_index:end),trajectory_y(start_index:end),control_time);
    thetar = interp1(trajectory_time(start_index:end),trajectory_heading(start_index:end),control_time);
    kappar = interp1(trajectory_time(start_index:end),trajectory_kappa(start_index:end),control_time);
    vr = interp1(trajectory_time(start_index:end),trajectory_speed(start_index:end),control_time);
    ar = interp1(trajectory_time(start_index:end),trajectory_accel(start_index:end),control_time);
else
    xr = trajectory_x(start_index);
    yr = trajectory_y(start_index);
    thetar = trajectory_heading(start_index);
    kappar = trajectory_kappa(start_index);
    vr = trajectory_speed(start_index);
    ar = trajectory_accel(start_index);
end

== matlab function EMPlanner_cs/Audi_A8_Sedan_1/control module2/control main/chassic steering system/MATLAB Function ==
  data: u input; right_steer output; la input; lb input
function right_steer = fcn(u,la,lb)
if abs(u)<1e-2
   right_steer = u;
else
   R =  (la+lb)/tan(u);
   right_steer = atan((la+lb)/(R+1.624/2));
end

== matlab function EMPlanner_cs/Audi_A8_Sedan_1/decision&planning module/EM Planner/calc plan start info and stitch trajectory1 ==
  data: pre_trajectory_x input; plan_start_x output; pre_trajectory_y input; pre_trajectory_heading input; pre_trajectory_kappa input; pre_trajectory_velocity input; pre_trajectory_accel input; pre_trajectory_time input; current_time input; host_x input; host_y input; host_heading_xy input; host_vx input; host_vy input; host_ax input; host_ay input; plan_start_y output; plan_start_heading output; plan_start_kappa output; plan_start_vx output; plan_start_vy output; plan_start_ax output; plan_start_ay output; plan_start_time output; stitch_x output; stitch_y output; stitch_heading output; stitch_kappa output; stitch_speed output; stitch_accel output; stitch_time output
function [plan_start_x,plan_start_y,plan_start_heading,plan_start_kappa,plan_start_vx,plan_start_vy,plan_start_ax,...
    plan_start_ay,plan_start_time,stitch_x,stitch_y,stitch_heading,stitch_kappa,stitch_speed,stitch_accel,stitch_time] ...
    = fcn(pre_trajectory_x,pre_trajectory_y,pre_trajectory_heading,pre_trajectory_kappa,pre_trajectory_velocity,...
    pre_trajectory_accel,pre_trajectory_time,current_time,host_x,host_y,host_heading_xy,host_vx,host_vy,host_ax,host_ay)
%该函数将计算规划的起点以及拼接轨迹的信息
%输入 上一周期的规划结果信息pre_trajectory x ,y,heading,kappa,velocity,accel,time
%     本周期的绝对时间current_time
%     定位信息host x,y,heading,kappa,vx,vy,ax,ay
%输出 规划起点信息plan_start x,y,heading,kappa,vx,vy,ax,ay(vx,vy,ax,ay)是世界坐标系的
%     待拼接的轨迹信息，一般在上一周期的轨迹中的current_time+100ms，往前取20个点。
%     当规划完成后，本周期的规划结果和stitch_trajectory一起拼好发给控制

%输出初始化
stitch_x = zeros(20,1);
stitch_y = zeros(20,1);
stitch_heading = zeros(20,1);
stitch_kappa = zeros(20,1);
stitch_speed = zeros(20,1);
stitch_accel = zeros(20,1);
%时间为负代表没有对应的拼接轨迹
stitch_time = ones(20,1)*-1;

%申明全局变量
persistent is_first_run;
if isempty(is_first_run)
    %代表代码首次运行
    is_first_run = 0;
    %按照轨迹拼接算法，应该用车辆动力学递推，但是首次运行车辆的速度都是0，所以没必要递推了
    plan_start_x = host_x;
    plan_start_y = host_y;
    plan_start_heading = host_heading_xy;
    plan_start_kappa = 0;
    plan_start_vx = 0;
    plan_start_vy = 0;
    plan_start_ax = 0;
    plan_start_ay = 0;
    %规划的起点的时间应该是当前时间+100ms
    plan_start_time = current_time + 0.1;
else
    %该函数不是首次运行
    x_cur = host_x;
    y_cur = host_y;
    heading_cur = host_heading_xy;
    kappa_cur = 0;
    %vx vy ax ay要转换成世界坐标系
    vx_cur = host_vx*cos(heading_cur) - host_vy*sin(heading_cur);
    vy_cur = host_vx*sin(heading_cur) + host_vy*cos(heading_cur);
    ax_cur = host_ax*cos(heading_cur) - host_ay*sin(heading_cur);
    ay_cur = host_ax*sin(heading_cur) + host_ay*cos(heading_cur);
    %规划周期
    dt = 0.1;
    %由于不是首次运行了，有上一时刻的轨迹了，找到上一周期轨迹规划的本周期车辆应该在的位置
    for i = 1:length(pre_trajectory_time) - 1
        if (pre_trajectory_time(i) <= current_time && pre_trajectory_time(i + 1) > current_time)
            break;
        end
    end
    %上一周期规划的本周期的车应该在的位置
    pre_x_desire = pre_trajectory_x(i);
    pre_y_desire = pre_trajectory_y(i);
    pre_heading_desire = pre_trajectory_heading(i);
    %计算横纵向误差
    %切向量
    tor = [cos(pre_heading_desire);sin(pre_heading_desire)];
    %法向量
    nor = [-sin(pre_heading_desire);cos(pre_heading_desire)];
    %误差向量
    d_err = [host_x;host_y] - [pre_x_desire;pre_y_desire];
    %纵向误差
    lon_err = abs(d_err'*tor);
    %横向误差
    lat_err = abs(d_err'*nor);
    %纵向误差大于2.5 横向误差大于0.5 认为控制没跟上
    if (lon_err > 2.5)||(lat_err > 0.5)
        %此分支处理控制未跟上的情况，规划起点通过运动学递推
        plan_start_x = x_cur + vx_cur * dt + 0.5 * ax_cur * dt * dt;
        plan_start_y = y_cur + vy_cur * dt + 0.5 * ay_cur * dt * dt;
        plan_start_vx = vx_cur + ax_cur * dt;
        plan_start_vy = vy_cur + ay_cur * dt;
        plan_start_heading = atan2(plan_start_vy,plan_start_vx);
        plan_start_ax = ax_cur;
        plan_start_ay = ay_cur;
        plan_start_kappa = kappa_cur;
        plan_start_time = current_time + 0.1;
        return;
    else
        %此分支表示控制能跟的上规划，开始拼接
        for j = i:length(pre_trajectory_time) - 1
            if (pre_trajectory_time(j) <= current_time + 0.1)&&(pre_trajectory_time(j + 1) > current_time + 0.1)
                break;
            end
        end
        %注：此算法要能运行需要trajectory的点有很高的密度
        plan_start_x = pre_trajectory_x(j);
        plan_start_y = pre_trajectory_y(j);
        plan_start_heading = pre_trajectory_heading(j);
        plan_start_kappa = pre_trajectory_kappa(j);
        %这里的pre_trajectory的速度,加速度是指轨迹的切向速度，切向加速度
        plan_start_vx = pre_trajectory_velocity(j) * cos(plan_start_heading);
        plan_start_vy = pre_trajectory_velocity(j) * sin(plan_start_heading);
        %pre_trajectory的加速度是切向加速度，要想计算ax,ay还要计算法向加速度
        %计算轨迹在current_time + 100ms 这个点的切向量法向量
        tor = [cos(plan_start_heading);sin(plan_start_heading)];
        nor = [-sin(plan_start_heading);cos(plan_start_heading)];
        a_tor = pre_trajectory_accel(j) * tor;
        a_nor = pre_trajectory_velocity(j)^2 * plan_start_kappa * nor ;
        plan_start_ax = a_tor(1) + a_nor(1);
        plan_start_ay = a_tor(2) + a_nor(2);
        plan_start_time = pre_trajectory_time(j);
        %计算拼接轨迹
        %j 表示 current_time + 0.1 的时间点在 pre_trajectory_time的编号
        %拼接是往从j开始，往前拼接20个，也就是pre_trajectory(j-1),j-2,j-3,....j-19
        %分两种情况，如果j小于20，意味着前面的轨迹点不够20个
        %如果j >= 20,意味着前面的点多于20个
        %还有一个细节需要考虑，pre_trajectory x(j) y(j) ....是规划的起点，那么在轨迹拼接时
        %需不需要在stitch_trajectory中把pre_trajectory x(j) y(j) ....包含进去
        %答案是否定的，不应该包进去，因为规划的起点会在规划模块计算完成后的结果中包含，如果在拼接的时候
        %还要包含，那就等于规划起点包含了两次
        %除非本周期计算的轨迹不包含规划起点，那么stitch_trajectory可以包含规划起点。
        %如果本周期计算的轨迹包含规划起点，那么stitch_trajectory就不可以包含规划起点。
        %我们选择规划包含起点，拼接不包含起点的做法
        
        %把起点去掉
        j = j - 1;
        if j >= 20
            stitch_x = pre_trajectory_x(j - 19:j);
            stitch_y = pre_trajectory_y(j - 19:j);
            stitch_heading = pre_trajectory_heading(j - 19:j);
            stitch_kappa = pre_trajectory_kappa(j - 19:j);
            stitch_speed = pre_trajectory_velocity(j - 19:j);
            stitch_accel = pre_trajectory_accel(j - 19:j);
            stitch_time = pre_trajectory_time(j - 19:j);
        else
            stitch_x(20 - j + 1:20) = pre_trajectory_x(1:j);
            stitch_y(20 - j + 1:20) = pre_trajectory_y(1:j);
            stitch_heading(20 - j + 1:20) = pre_trajectory_heading(1:j);
            stitch_kappa(20 - j + 1:20) = pre_trajectory_kappa(1:j);
            stitch_speed(20 - j + 1:20) = pre_trajectory_velocity(1:j);
            stitch_accel(20 - j + 1:20) = pre_trajectory_accel(1:j);
            stitch_time(20 - j + 1:20) = pre_trajectory_time(1:j);           
        end   
    end    
end

== matlab function EMPlanner_cs/Audi_A8_Sedan_1/decision&planning module/EM Planner/genrate index to s ==
  data: path_x_set_gcs input; matchPoint_index_s_set_fcs output; path_y_set_gcs input; path_heading_set_gcs input; origin_match_point_index input; origin_point_x_gcs input; origin_point_y_gcs input
function matchPoint_index_s_set_fcs = fun(path_x_set_gcs,path_y_set_gcs,path_heading_set_gcs,...
    origin_match_point_index,origin_point_x_gcs,origin_point_y_gcs)
% 该函数将以给定路径采样点为s轴 取自身在给定路径上投影点作为坐标原点 来求出每个采样点编号和对应s坐标的集合
% path_x_set_gcs,path_y_set_gcs 给定路径采样点集合
% origin_match_point_index,origin_point_x_gcs,origin_point_y_gcs   坐标原点信息
% 输出初始化
matchPoint_index_s_set_fcs = zeros(length(path_x_set_gcs),1);
% 首先给定路径采样点每个点到第一个采样点的弧长
for i = 2:length(path_x_set_gcs)
    dis = sqrt((path_x_set_gcs(i)-path_x_set_gcs(i-1))^2+(path_y_set_gcs(i)-path_y_set_gcs(i-1))^2); % 以直线代替相邻点弧长
    matchPoint_index_s_set_fcs(i) = dis + matchPoint_index_s_set_fcs(i-1); % 累加得到
end
%再求出坐标原点到第一个采样点的弧长
s = CalSFromOriginPoint(matchPoint_index_s_set_fcs,path_x_set_gcs,path_y_set_gcs,path_heading_set_gcs,...
                            origin_point_x_gcs,origin_point_y_gcs,origin_match_point_index);
% 得到每个采样点到坐标原点的弧长对应关系 亦即真正的s坐标对应编号关系
matchPoint_index_s_set_fcs = matchPoint_index_s_set_fcs - ones(length(path_x_set_gcs),1)*s;
end

== stateflow chart EMPlanner_cs/Audi_A8_Sedan_1/Chart ==
  (default) -> (junction 5)
  (junction 5) -> (junction 7)
  (junction 7) -> (junction 9) [order 1] : [i >= 100]
  (junction 7) -> (junction 13) [order 2] : {
      | i = i + 1;
      | }
  (junction 9) -> (junction 11) : {
      | do_planning;
      | i = 1;
      | }
  (junction 11) -> (junction 13)
  (junction 13) -> (junction 16)
  (junction 16) -> (junction 18) [order 1] : [j >= 10]
  (junction 16) -> (junction 22) [order 2] : {
      | j = j + 1;
      | }
  (junction 18) -> (junction 20) : {
      | do_control;
      | j = 1;
      | }
  (junction 20) -> (junction 22)
  (junction 22) -> (junction 25)
  data: i local =1; j local =1
  events: do_planning output FUNCTION_CALL_EVENT; do_control output FUNCTION_CALL_EVENT

== matlab function EMPlanner_cs/Audi_A8_Sedan_1/decision&planning module/EM Planner/Cartesian2Frenet/MATLAB Function3 ==
  data: l_set input; s_dot_set output; vx_set input; vy_set input; proj_heading_set input; proj_kappa_set input; l_dot_set output; dl_set output
function [s_dot_set,l_dot_set,dl_set] = fcn(l_set,vx_set,vy_set,proj_heading_set,proj_kappa_set)
%该函数将计算frenet坐标系下的s_dot, l_dot, dl/ds
n = 128;
% 输出初始化
s_dot_set = ones(n,1)*nan;
l_dot_set = ones(n,1)*nan;
dl_set = ones(n,1)*nan;

for i = 1 : length(l_set)
    if isnan(l_set(i))
        break;
    end
    v_h = [vx_set(i);vy_set(i)];
    n_r = [-sin(proj_heading_set(i));cos(proj_heading_set(i))];
    t_r = [cos(proj_heading_set(i));sin(proj_heading_set(i))];
    l_dot_set(i) = v_h'*n_r;
    s_dot_set(i) = v_h'*t_r/(1 - proj_kappa_set(i)*l_set(i));
    %%%向量法做cartesian与frenet的转换要更简单，但是也有缺点，向量法必须依赖速度加速度
    %l' = l_dot/s_dot 但是如果s_dot = 0 此方法就失效了
    if abs(s_dot_set(i)) < 1e-6
        dl_set(i) = 0;
    else
        dl_set(i) = l_dot_set(i)/s_dot_set(i);
    end
end

== matlab function EMPlanner_cs/Audi_A8_Sedan_1/decision&planning module/EM Planner/Cartesian2Frenet/MATLAB Function ==
  data: x_set_gcs input; s_set_fcs output; y_set_gcs input; path_x_set_gcs input; path_y_set_gcs input; path_heading_set_gcs input; match_point_index_set input; proj_point_x_set_gcs input; proj_point_y_set_gcs input; proj_point_heading_set_gcs input; l_set_fcs output; matchPoint_index_s_set_fcs input
function [s_set_fcs,l_set_fcs] = fun(x_set_gcs,y_set_gcs,path_x_set_gcs,path_y_set_gcs,path_heading_set_gcs,match_point_index_set,...
    proj_point_x_set_gcs,proj_point_y_set_gcs,proj_point_heading_set_gcs,matchPoint_index_s_set_fcs)
% 将函数批量将给定点的(x,y)转化成(s,l)
% 假设最多有181个点需要转换坐标
n = 181;
% 输出初始化
s_set_fcs = ones(n,1)*nan; l_set_fcs = ones(n,1)*nan;
for i = 1:length(x_set_gcs)
    if isnan(x_set_gcs(i))
        break;
    end
    s_set_fcs(i) = CalSFromOriginPoint(matchPoint_index_s_set_fcs,path_x_set_gcs,path_y_set_gcs,path_heading_set_gcs,...
                                proj_point_x_set_gcs(i),proj_point_y_set_gcs(i),match_point_index_set(i));
    vector_rh = [x_set_gcs(i),y_set_gcs(i)];
    vector_rp = [proj_point_x_set_gcs(i),proj_point_y_set_gcs(i)];
    vector_np = [-sin(proj_point_heading_set_gcs(i)),cos(proj_point_heading_set_gcs(i))];
    l_set_fcs(i) = dot(vector_rh-vector_rp, vector_np);
end
end

== matlab function EMPlanner_cs/Audi_A8_Sedan_2/PathFollower_Preview_1/LateralController/Calculate delta steering error/eml_delta_steering_error ==
  data: v_x_vehicle input; v_x_vehicle_Min input; t_Preview_LatCtrl input; delta_steeringwheeltotal output; v_y_vehicle input; yawrate_vehicle input; CorneringStiffness_Tyres_Front input; CorneringStiffness_Tyres_Rear input; m_vehicle_total input; inertia_z_vehicle_total input; e_Lat input size=10; Pos_x_CoG_Vehicle input; wheelbase input; RefreshCounter parameter
function delta_steeringwheeltotal = eml_delta_steering_error(v_x_vehicle,v_x_vehicle_Min,t_Preview_LatCtrl,v_y_vehicle,yawrate_vehicle,CorneringStiffness_Tyres_Front,CorneringStiffness_Tyres_Rear,m_vehicle_total,inertia_z_vehicle_total,e_Lat,Pos_x_CoG_Vehicle,wheelbase,RefreshCounter)

delta_steeringwheeltotal = emlfcn_delta_steering_error(v_x_vehicle,v_x_vehicle_Min,t_Preview_LatCtrl,v_y_vehicle,yawrate_vehicle,CorneringStiffness_Tyres_Front,CorneringStiffness_Tyres_Rear,m_vehicle_total,inertia_z_vehicle_total,e_Lat,Pos_x_CoG_Vehicle,wheelbase,RefreshCounter);

% end function
